simulink model "model2"  (R2021b)
settings: Solver=FixedStepAuto  StartTime=0.0  StopTime=10.0  FixedStep=0.001  RelTol=1e-3
undefined symbols (not defined in the file): DiscIntNeverNeededParam
libraries: simulink x3
settings Model: Creator=O  LastModifiedBy=wangzixuan

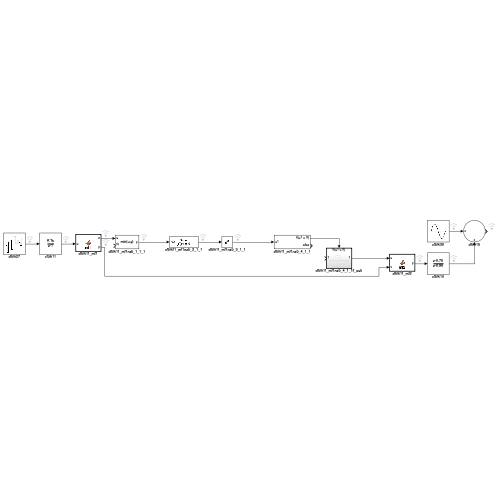
[thumbnail: Simulink's stored preview of the top-level diagram]
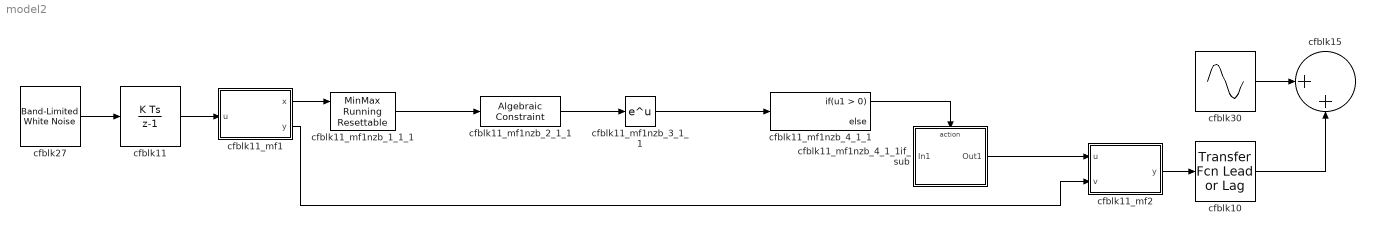
== system model2 ==
  cfblk10 : simulink/Discrete/Transfer Fcn Lead or Lag  PoleZ=0.95  ZeroZ=0.75  ICPrevOutput=0.0  ICPrevInput=0.0  DoSatur=off
      settings: SourceProductBaseCode=SL
  cfblk11 : DiscreteIntegrator  OutDataTypeStr=double  ICPrevOutput=DiscIntNeverNeededParam  ICPrevScaledInput=DiscIntNeverNeededParam
  cfblk11_mf1 : MATLAB Function  TreatAsAtomicUnit=on
  cfblk11_mf1nzb_1_1_1 : simulink/Math Operations/MinMax Running Resettable  Function=min  vinit=0.0
  cfblk11_mf1nzb_2_1_1 : AlgebraicConstraint
  cfblk11_mf1nzb_3_1_1 : Math  SaturateOnIntegerOverflow=on
  cfblk11_mf1nzb_4_1_1 : If
  cfblk11_mf1nzb_4_1_1if_sub : Subsystem  TreatAsAtomicUnit=on
  cfblk11_mf2 : MATLAB Function  TreatAsAtomicUnit=on
  cfblk15 : Sum  Inputs=|++  OutDataTypeStr=double
  cfblk27 : simulink/Sources/Band-Limited White Noise  Cov=[7496925313.772144]  Ts=0.1  seed=[9446467060.000000]
  cfblk30 : Sin  Amplitude=[-484213518.220894]  Bias=[-227187939.059104]  SampleTime=0
  wires:
  cfblk11_mf1nzb_1_1_1/1 -> cfblk11_mf1nzb_2_1_1/1
  cfblk11/1 -> cfblk11_mf1/1(u)
  cfblk11_mf1nzb_4_1_1if_sub/1(Out1) -> cfblk11_mf2/1(u)
  cfblk30/1 -> cfblk15/1
  cfblk11_mf1/2(y) -> cfblk11_mf2/2(v)
  cfblk11_mf1/1(x) -> cfblk11_mf1nzb_1_1_1/1
  cfblk11_mf1nzb_3_1_1/1 -> cfblk11_mf1nzb_4_1_1/1
  cfblk11_mf1nzb_2_1_1/1 -> cfblk11_mf1nzb_3_1_1/1
  cfblk10/1 -> cfblk15/2
  cfblk11_mf2/1(y) -> cfblk10/1
  cfblk27/1 -> cfblk11/1
  cfblk11_mf1nzb_4_1_1/1 -> cfblk11_mf1nzb_4_1_1if_sub/Action

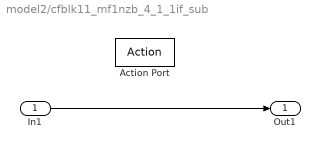
== system model2/cfblk11_mf1nzb_4_1_1if_sub ==
  In1 : Inport
  Action Port : ActionPort  ActionPortLabel=if(u1 > 0)
  Out1 : Outport
  wires:
  In1/1 -> Out1/1

== matlab function model2/cfblk11_mf2 ==
  data: u input; y output; v input
function y = mf2(u,v)
y = v;
end

== matlab function model2/cfblk11_mf1 ==
  data: x output; u input; y output
function [x,y]= mf1(u)
x = u;
y = u;
end
